simulink model "exampleEvaporation_Enthalpy"  (R2018b)
settings: Solver=ode45  StartTime=0.0  StopTime=10.0  RelTol=1e-3  EnableMultiTasking=on
libraries: carnot x4
settings Model: Creator=drhf  LastModifiedBy=drhf
settings DataIOCC: LimitDataPoints=on  SaveFormat=Array  SignalLoggingSaveFormat=ModelDataLogs
settings OptimizationCC: ExpressionDepthLimit=2147483647  LifeSpan=inf
settings DebuggingCC: UnderspecifiedInitializationDetection=Classic  MergeDetectMultiDrivingBlocksExec=none  SolverPrmCheckMsg=warning  StateNameClashWarn=warning  SFUnexpectedBacktrackingDiag=warning  SFNoUnconditionalDefaultTransitionDiag=warning  SFExecutionAtInitializationDiag=none
settings HardwareCC: ProdBitPerPointer=32  ProdBitPerSizeT=32  ProdBitPerPtrDiffT=32  ProdLargestAtomicFloat=None  ProdIntDivRoundTo=Undefined  ProdEndianess=Unspecified  ProdWordSize=32  ProdHWDeviceType=32-bit Generic
settings ModelReferenceCC: PropagateSignalLabelsOutOfModel=off
settings SFSimCC: SimUseLocalCustomCode=off
settings RTWCC: RTWUseLocalCustomCode=off
settings CodeAppCC: StateflowObjectComments=on
settings GRTTargetCC: TargetLangStandard=C89/C90 (ANSI)  GeneratePreprocessorConditionals=Disable all  CombineOutputUpdateFcns=off  GRTInterface=on
settings ConfigComp: CovMetricSettings=dw  CovHtmlReporting=on  CovSaveCumulativeToWorkspaceVar=on  CovSaveSingleToWorkspaceVar=on  CovExternalEMLEnable=off

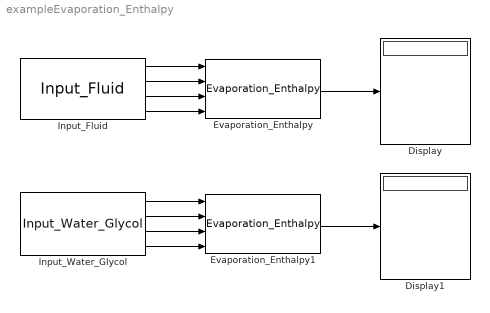
== system exampleEvaporation_Enthalpy ==
  Display : Display
  Display1 : Display
  Evaporation_Enthalpy : carnot/Basic/Material_Properties/Evaporation_Enthalpy  VariantControl=CarlibClassic  INPUTARGUMENTS=state variables (classic)  DEBUGLEVEL=WARNINGLEVEL  MAXTOTALMESSAGES=inf  MAXCONSECUTIVEMESSAGES=inf  WRITETOFILE=0  FILENAME='errors.txt'
  Evaporation_Enthalpy1 : carnot/Basic/Material_Properties/Evaporation_Enthalpy  VariantControl=CarlibClassic  INPUTARGUMENTS=state variables (classic)  DEBUGLEVEL=WARNINGLEVEL  MAXTOTALMESSAGES=inf  MAXCONSECUTIVEMESSAGES=inf  WRITETOFILE=0  FILENAME='errors.txt'
  Input_Fluid : carnot/Basic/Material_Properties/Input_Fluid  fluid=Water  T=[10:10:50]  p=1e5  x=0.005
  Input_Water_Glycol : carnot/Basic/Material_Properties/Input_Water_Glycol  T=20  p=1e5  g=0.4
  wires:
  Input_Fluid/1 -> Evaporation_Enthalpy/1
  Input_Fluid/2 -> Evaporation_Enthalpy/2
  Input_Fluid/3 -> Evaporation_Enthalpy/3
  Input_Fluid/4 -> Evaporation_Enthalpy/4
  Evaporation_Enthalpy/1 -> Display/1
  Input_Water_Glycol/1 -> Evaporation_Enthalpy1/1
  Input_Water_Glycol/2 -> Evaporation_Enthalpy1/2
  Input_Water_Glycol/3 -> Evaporation_Enthalpy1/3
  Input_Water_Glycol/4 -> Evaporation_Enthalpy1/4
  Evaporation_Enthalpy1/1 -> Display1/1
